simulink model "IMU_Serial_Example"  (R2012b)
settings: Solver=FixedStepDiscrete  SolverMode=SingleTasking  StartTime=0.0  StopTime=10.0  RelTol=1e-3
libraries: Timing_Library x2, IMU_Library x1, Serial_Library x1
settings Model: ExtModeTrigDuration=2  Creator=Hugon  LastModifiedBy=Hugon
settings OptimizationCC: OptimizeModelRefInitCode=on  LifeSpan=1
settings DebuggingCC: SolverPrmCheckMsg=none  StrictBusMsg=Warning
settings HardwareCC: ProdBitPerInt=16  ProdBitPerPointer=8  ProdIntDivRoundTo=Zero  ProdEndianess=LittleEndian  ProdWordSize=8  ProdHWDeviceType=Atmel->AVR
settings RTWCC: SystemTargetFile=realtime.tlc  GenerateMakefile=off  TemplateMakefile=realtime.tmf  Description=Real-Time Toolbox  RTWVerbose=off  ProcessScript=realtime_make_rtw_hook
settings STFCustomTargetCC: TargetLibSuffix=.a  CodeReplacementLibrary=ANSI_C  GenerateSampleERTMain=on  ERTCustomFileBanners=on  SupportNonInlinedSFcns=off  SupportVariableSizeSignals=on  GRTInterface=off  SystemTargetFile=realtime.tlc
settings ERTTargetCC: CodeReplacementLibrary=ANSI_C  MultiwordLength=2048  GenerateSampleERTMain=on  ParMdlRefBuildCompliant=off  CompOptLevelCompliant=off  ConcurrentExecutionCompliant=off  CombineOutputUpdateFcns=off  ERTFirstTimeCompliant=off  SupportContinuousTime=on  SupportVariableSizeSignals=on  ModelStepFunctionPrototypeControlCompliant=off  CPPClassGenCompliant=off  ExtModeTransport=3  ExtModeMexFile=ext_serial_win32_comm  ExtModeMexArgs=0 1 9600  InlinedParameterPlacement=NonHierarchical  ERTSrcFileBannerTemplate=realtime_code_template.cgt  ERTHdrFileBannerTemplate=realtime_code_template.cgt  ERTDataSrcFileTemplate=realtime_code_template.cgt  ERTDataHdrFileTemplate=realtime_code_template.cgt  ERTCustomFileTemplate=realtime_file_process.tlc  ConvertIfToSwitch=off  SuppressUnreachableDefaultCases=off

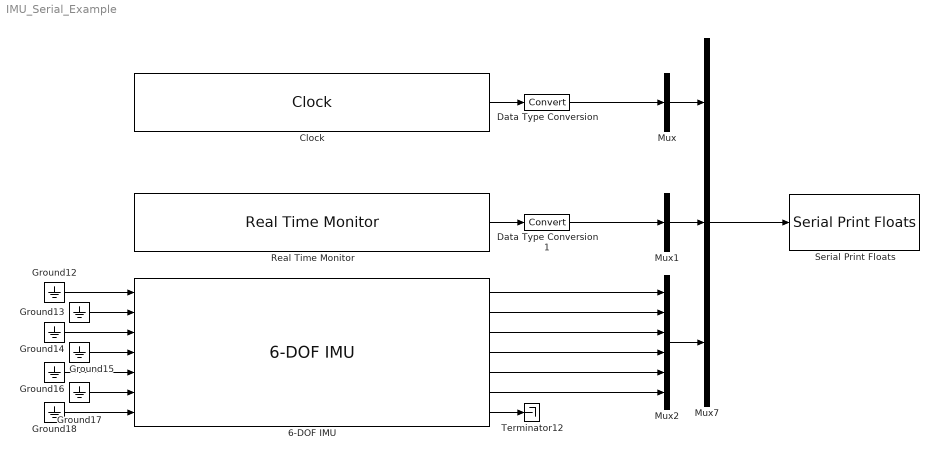
== system IMU_Serial_Example ==
  6-DOF IMU : IMU_Library/6-DOF IMU  lpf_filt_freq_hz_ix=20 Hz  gyro_scale_ix=+/- 500 deg/sec  accel_scale_ix=+/- 8g  SampleTime=0.02  lpf_filt_freq_hz=5 Hz  gyro_scale=+/- 250 deg/sec  accel_scale=+/- 2g
  Clock : Timing_Library/Clock  SampleTime=.02
  Data Type Conversion : DataTypeConversion
  Data Type Conversion1 : DataTypeConversion
  Ground{12..18} (7 alike) : Ground
  Mux : Mux  Inputs=1
  Mux1 : Mux  Inputs=1
  Mux2 : Mux  Inputs=6
  Mux7 : Mux  Inputs=3
  Real Time Monitor : Timing_Library/Real Time Monitor  SampleTime=0.02
  Serial Print Floats : Serial_Library/Serial Print Floats  baud=57600  uart=UART0  SampleTime=-1
  Terminator12 : Terminator
  wires:
  Mux7/1 -> Serial Print Floats/1
  Clock/1 -> Data Type Conversion/1
  Real Time Monitor/1 -> Data Type Conversion1/1
  6-DOF IMU/1 -> Mux2/1
  6-DOF IMU/2 -> Mux2/2
  6-DOF IMU/3 -> Mux2/3
  6-DOF IMU/4 -> Mux2/4
  6-DOF IMU/5 -> Mux2/5
  6-DOF IMU/6 -> Mux2/6
  Mux/1 -> Mux7/1
  Mux1/1 -> Mux7/2
  Mux2/1 -> Mux7/3
  6-DOF IMU/7 -> Terminator12/1
  Ground12/1 -> 6-DOF IMU/1
  Ground13/1 -> 6-DOF IMU/2
  Ground14/1 -> 6-DOF IMU/3
  Ground15/1 -> 6-DOF IMU/4
  Ground16/1 -> 6-DOF IMU/5
  Ground17/1 -> 6-DOF IMU/6
  Ground18/1 -> 6-DOF IMU/7
  Data Type Conversion/1 -> Mux/1
  Data Type Conversion1/1 -> Mux1/1
